simulink model "compute_thruster_misalignment_mc"  (R2013b)
settings: Solver=FixedStepDiscrete  StartTime=0.0  StopTime=1  FixedStep=1  RelTol=1e-3
undefined symbols (not defined in the file or in its folder): q_thr_to_zthr, qxrot, qzrot, thr_unit
libraries: util_quat_lib x6, util_common_lib x2
settings Model: Creator=Jim Kaidy  LastModifiedBy=jkaidy
settings DataIOCC: SignalLoggingSaveFormat=ModelDataLogs
settings DebuggingCC: AlgebraicLoopMsg=error  ArtificialAlgebraicLoopMsg=error

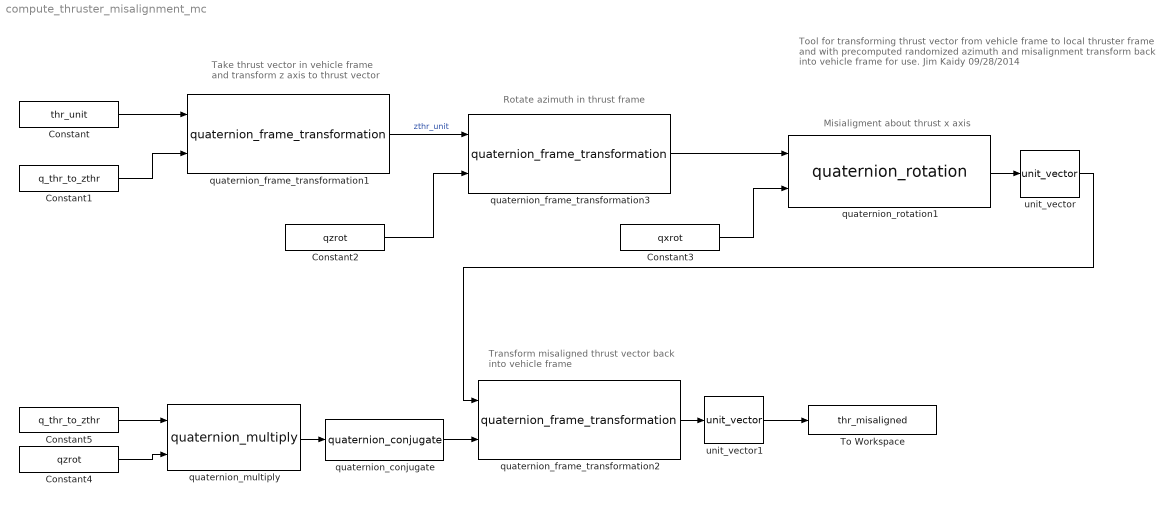
== system compute_thruster_misalignment_mc ==
  note: Tool for transforming thrust vector from vehicle frame to local thruster frame
      | and with precomputed randomized azimuth and misalignment transform
      | back into vehicle frame for use.
      | Jim Kaidy 09/28/2014
  note: Transform misaligned thrust vector back
      |  into vehicle frame
  note: Misialigment about thrust x axis
  note: Rotate azimuth in thrust frame
  note: Take thrust vector in vehicle frame
      | and transform z axis to thrust vector
  Constant : Constant  Value=thr_unit
  Constant1 : Constant  Value=q_thr_to_zthr
  Constant2 : Constant  Value=qzrot
  Constant3 : Constant  Value=qxrot
  Constant4 : Constant  Value=qzrot
  Constant5 : Constant  Value=q_thr_to_zthr
  To Workspace : ToWorkspace  VariableName=thr_misaligned  SampleTime=-1  SaveFormat=Timeseries
  quaternion_conjugate : util_quat_lib/quaternion_conjugate  SystemSampleTime=-1
  quaternion_frame_transformation1 : util_quat_lib/quaternion_frame_transformation  SystemSampleTime=-1
  quaternion_frame_transformation2 : util_quat_lib/quaternion_frame_transformation  SystemSampleTime=-1
  quaternion_frame_transformation3 : util_quat_lib/quaternion_frame_transformation  SystemSampleTime=-1
  quaternion_multiply : util_quat_lib/quaternion_multiply  SystemSampleTime=-1
  quaternion_rotation1 : util_quat_lib/quaternion_rotation  SystemSampleTime=-1
  unit_vector : util_common_lib/unit_vector  SystemSampleTime=-1
  unit_vector1 : util_common_lib/unit_vector  SystemSampleTime=-1
  wires:
  Constant/1 -> quaternion_frame_transformation1/1
  Constant1/1 -> quaternion_frame_transformation1/2
  Constant2/1 -> quaternion_frame_transformation3/2
  quaternion_frame_transformation1/1 -> quaternion_frame_transformation3/1  "zthr_unit"
  Constant3/1 -> quaternion_rotation1/2
  quaternion_rotation1/1 -> unit_vector/1
  quaternion_frame_transformation3/1 -> quaternion_rotation1/1
  unit_vector/1 -> quaternion_frame_transformation2/1
  quaternion_frame_transformation2/1 -> unit_vector1/1
  unit_vector1/1 -> To Workspace/1
  quaternion_conjugate/1 -> quaternion_frame_transformation2/2
  Constant4/1 -> quaternion_multiply/2
  Constant5/1 -> quaternion_multiply/1
  quaternion_multiply/1 -> quaternion_conjugate/1
